simulink model "Heating"  (Simulink 8.1)
settings: Solver=ode45  StartTime=0.0  StopTime=1  RelTol=1e-3
values from neighbouring files (symbols this model uses):
  boiler = collect(4,1)    [run.m]
  chp1 = collect(2,1)    [run.m]
  chp2 = collect(3,1)    [run.m]
  Ecth = Eth    [run.m]
  Pch = collect(6,1)    [run.m]
  Pre = collect(5,1)    [run.m]
  stunde = stunde+1    (= 2401)    [run.m]
settings Model: Creator=Ming  LastModifiedBy=Ming
settings DataIOCC: SignalLoggingSaveFormat=Dataset
settings OptimizationCC: ExpressionDepthLimit=128
settings DebuggingCC: FcnCallInpInsideContextMsg=EnableAllAsError
settings GRTTargetCC: CombineOutputUpdateFcns=on  GRTInterface=off

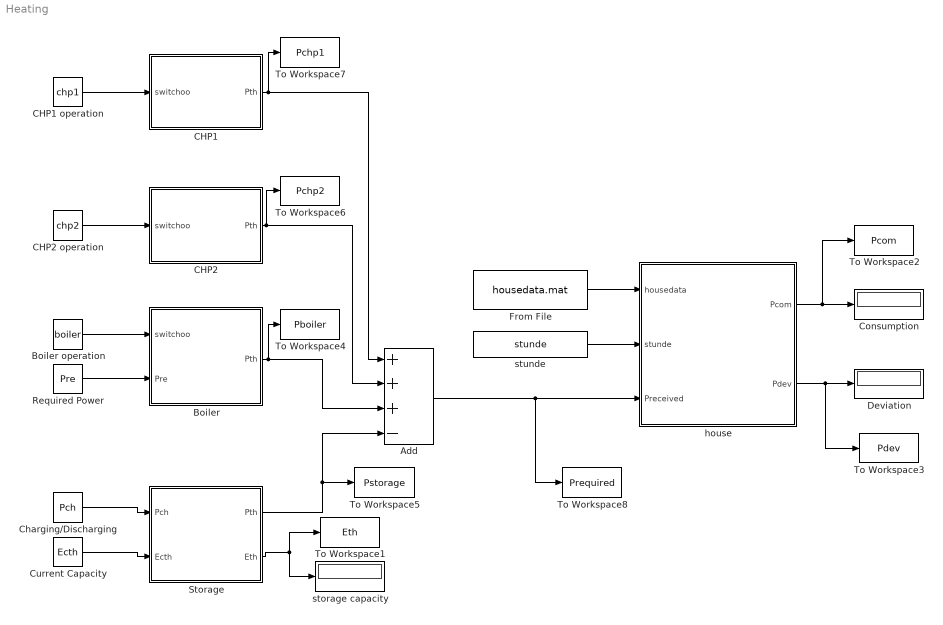
== system Heating ==
  Add : Sum  Inputs=+++-
  Boiler : MATLAB Function  TreatAsAtomicUnit=on
  Boiler operation : Constant  Value=boiler
  CHP1 : MATLAB Function  TreatAsAtomicUnit=on
  CHP1 operation : Constant  Value=chp1
  CHP2 : MATLAB Function  TreatAsAtomicUnit=on
  CHP2 operation : Constant  Value=chp2
  Charging/Discharging : Constant  Value=Pch
  Consumption : Display
  Current Capacity : Constant  Value=Ecth
  Deviation : Display
  From File : FromFile  FileName=housedata.mat  OutDataTypeStr=double  SampleTime=0
  Required Power : Constant  Value=Pre
  Storage : MATLAB Function  TreatAsAtomicUnit=on
  To Workspace1 : ToWorkspace  VariableName=Eth  SampleTime=-1
      settings: LoadFcn=send
  To Workspace2 : ToWorkspace  VariableName=Pcom  SampleTime=-1
  To Workspace3 : ToWorkspace  VariableName=Pdev  SampleTime=-1
  To Workspace4 : ToWorkspace  VariableName=Pboiler  SampleTime=-1
  To Workspace5 : ToWorkspace  VariableName=Pstorage  SampleTime=-1
  To Workspace6 : ToWorkspace  VariableName=Pchp2  SampleTime=-1
  To Workspace7 : ToWorkspace  VariableName=Pchp1  SampleTime=-1
      settings: StopFcn=callback
  To Workspace8 : ToWorkspace  VariableName=Prequired  SampleTime=-1
  house : MATLAB Function  TreatAsAtomicUnit=on
  storage capacity : Display
  stunde : Constant  Value=stunde
  wires:
  CHP1 operation/1 -> CHP1/1(switchoo)
  Boiler operation/1 -> Boiler/1(switchoo)
  Required Power/1 -> Boiler/2(Pre)
  Charging/Discharging/1 -> Storage/1(Pch)
  CHP2 operation/1 -> CHP2/1(switchoo)
  From File/1 -> house/1(housedata)
  house/1(Pcom) -> To Workspace2/1, Consumption/1
  stunde/1 -> house/2(stunde)
  Boiler/1(Pth) -> To Workspace4/1, Add/3
  Storage/1(Pth) -> To Workspace5/1, Add/4
  CHP2/1(Pth) -> To Workspace6/1, Add/2
  CHP1/1(Pth) -> To Workspace7/1, Add/1
  Add/1 -> To Workspace8/1, house/3(Preceived)
  house/2(Pdev) -> To Workspace3/1, Deviation/1
  Current Capacity/1 -> Storage/2(Ecth)
  Storage/2(Eth) -> storage capacity/1, To Workspace1/1

== matlab function Boiler ==
  data: switchoo input double; Pth output double; Pre input double
function Pth = Boiler(switchoo, Pre)
%#codegen
 if switchoo==1 
     Pth=Pre;
 else
     Pth=0;  

 end

== matlab function CHP1 ==
  data: switchoo input double; Pth output double
function Pth = CHP1(switchoo)
%#codegen
Pmax=2.155;
 if switchoo==1 
     Pth=Pmax;
 else 
     Pth=0;  
     
 end

== matlab function Storage ==
  data: Pth output double; Pch input double; Eth output double; Ecth input double
function [Pth, Eth]= Storage(Pch, Ecth)
%#codegen
%Eth=Peth;
tsam=1;

Eth= Ecth+(Pch)*tsam;  

Pth=Pch;
 

end

== matlab function house ==
  data: housedata input double; Pcom output double; stunde input double; Preceived input double; Pdev output double
function [Pcom, Pdev] = household(housedata,stunde, Preceived)
%#codegen
 
Pcom=housedata(stunde,1);
Pdev=Preceived-Pcom;
%     Pcom=DataReceived(1,1);

end

== matlab function CHP2 ==
  data: switchoo input double; Pth output double
function Pth = CHP2(switchoo)
%#codegen
Pmax=2.155;
 if switchoo==1 
     Pth=Pmax;
 else 
     Pth=0;  
     
 end
